simulink model "differential_eq"  (R2019a)
settings: Solver=ode45  StartTime=0.0  StopTime=10.0  RelTol=1e-3
settings Model: Creator=INDIA  LastModifiedBy=INDIA

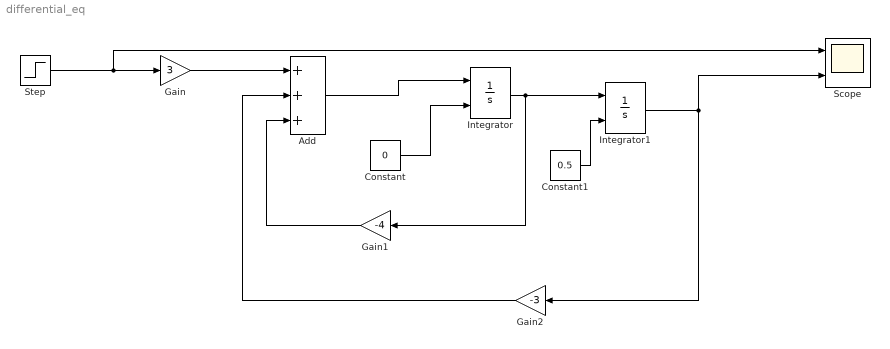
== system differential_eq ==
  Add : Sum  Inputs=+++
  Constant : Constant  Value=0
  Constant1 : Constant  Value=0.5
  Gain : Gain  Gain=3
  Gain1 : Gain  Gain=-4
  Gain2 : Gain  Gain=-3
  Integrator : Integrator  InitialConditionSource=external
  Integrator1 : Integrator  InitialConditionSource=external
  Scope : Scope  NumInputPorts=2
  Step : Step  SampleTime=0
  wires:
  Gain/1 -> Add/1
  Step/1 -> Scope/1, Gain/1
  Add/1 -> Integrator/1
  Integrator/1 -> Gain1/1, Integrator1/1
  Constant1/1 -> Integrator1/2
  Constant/1 -> Integrator/2
  Integrator1/1 -> Scope/2, Gain2/1
  Gain1/1 -> Add/3
  Gain2/1 -> Add/2
